simulink model "gps_estimate_pointsolution_demo"  (Simulink 7.3)
settings: Solver=ode45  StartTime=0.0  StopTime=86400  RelTol=1e-3
undefined symbols (not defined in the file): WGS
libraries: rapidstm32_gps_lib x6
settings Model: Creator=Compaq  LastModifiedBy=Compaq

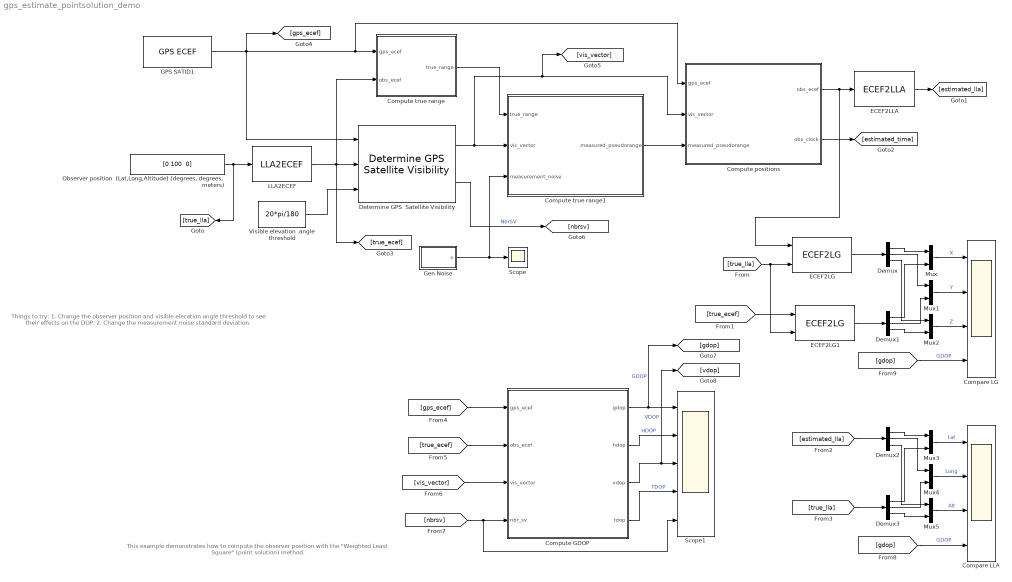
== system gps_estimate_pointsolution_demo ==
  note: This example demonstrates how to compute the observer position
      | with the "Weighted Least Square" (point solution) method.
  note: Things to try:
      | 1. Change the observer position and visible elecation angle threshold
      | to see their effects on the DOP.
      | 2. Change the measurement noise standard deviation.
  Compare LG : Scope  NumInputPorts=4
      settings: TimeRange=35000  YMin=-300~-400~-6.37925e+006~1.3  YMax=350~350~-6.377e+006~2  MaxDataPoints=1000
  Compare LLA : Scope  NumInputPorts=4
      settings: YMin=-0.00025~99.9995~-100~1.3  YMax=0.00025~100~100~1.95  SaveName=ScopeData2  MaxDataPoints=1000
  Compute GDOP : Stateflow chart
  Compute positions : Stateflow chart
  Compute true range : Stateflow chart
  Compute true range1 : Stateflow chart
  Demux{,1..3} (4 alike) : Demux  Outputs=3
  Determine GPS  Satellite Visibility : rapidstm32_gps_lib/Determine GPS  Satellite Visibility
  ECEF2LG : rapidstm32_gps_lib/ECEF2LG  lgoutput_format=NED  latlong_format=Degrees
  ECEF2LG1 : rapidstm32_gps_lib/ECEF2LG  lgoutput_format=NED  latlong_format=Degrees
  ECEF2LLA : rapidstm32_gps_lib/ECEF2LLA  latlong_format=Degrees  altitude_format=Meters  refellipsoid=WGS-84  re=6378137  epsilon=0.081819190842622
  GPS SATID1 : rapidstm32_gps_lib/GPS ECEF  satid=All 24  t0=0  sampletime=30
  Gen Noise : Stateflow chart
  LLA2ECEF : rapidstm32_gps_lib/LLA2ECEF  latlong_format=Degrees  refellipsoid=WGS-84  re=6378137  epsilon=0.081819190842622
  Mux{,1..5} (6 alike) : Mux  Inputs=2
  "Observer position  (Lat,Long,Altitude) (degrees, degrees, meters)" : Constant  Value="[0 100  0]"  OutDataType=fixdt(1, 16)  OutScaling=2^0
  Scope : Scope
      settings: YMin=-35  YMax=40  MaxDataPoints=1000
  Scope1 : Scope  NumInputPorts=5
      settings: TimeRange=86400  YMin=1~0~0~-8.67362e-019~1  YMax=8~30~25~0.03~4  SaveName=ScopeData3
  Visible elevation  angle threshold : Constant  Value=20*pi/180  OutDataType=fixdt(1, 16)  OutScaling=2^0
  wires:
  GPS SATID1/1 -> Determine GPS  Satellite Visibility/1, Compute true range/1(gps_ecef), Compute positions/1(gps_ecef), [gps_ecef]
  "Observer position  (Lat,Long,Altitude) (degrees, degrees, meters)"/1 -> LLA2ECEF/1, [true_lla]
  LLA2ECEF/1 -> Compute true range/2(obs_ecef), Determine GPS  Satellite Visibility/2, [true_ecef]
  Visible elevation  angle threshold/1 -> Determine GPS  Satellite Visibility/3
  Compute true range/1(true_range) -> Compute true range1/1(true_range)
  Determine GPS  Satellite Visibility/1 -> Compute true range1/2(vis_vector), Compute positions/2(vis_vector), [vis_vector]
  Gen Noise/1(n) -> Scope/1, Compute true range1/3(measurement_noise)
  Compute true range1/1(measured_pseudorange) -> Compute positions/3(measured_pseudorange)
  Determine GPS  Satellite Visibility/2 -> [nbrsv]  "NbrSV"
  Compute positions/1(obs_ecef) -> ECEF2LLA/1, ECEF2LG/1
  ECEF2LLA/1 -> [estimated_lla]
  Compute positions/2(obs_clock) -> [estimated_time]
  [true_lla] -> ECEF2LG/2, ECEF2LG1/2
  [true_ecef] -> ECEF2LG1/1
  ECEF2LG/1 -> Demux/1
  ECEF2LG1/1 -> Demux1/1
  Mux/1 -> Compare LG/1  "X"
  Mux1/1 -> Compare LG/2  "Y"
  Mux2/1 -> Compare LG/3  "Z"
  Demux/1 -> Mux/1
  Demux1/1 -> Mux/2
  Demux/2 -> Mux1/1
  Demux1/2 -> Mux1/2
  Demux/3 -> Mux2/1
  Demux1/3 -> Mux2/2
  Mux3/1 -> Compare LLA/1  "Lat"
  Mux4/1 -> Compare LLA/2  "Long"
  Mux5/1 -> Compare LLA/3  "Alt"
  Demux2/1 -> Mux3/1
  Demux3/1 -> Mux3/2
  Demux2/2 -> Mux4/1
  Demux3/2 -> Mux4/2
  Demux2/3 -> Mux5/1
  Demux3/3 -> Mux5/2
  [true_lla] -> Demux3/1
  [estimated_lla] -> Demux2/1
  Compute GDOP/1(gdop) -> Scope1/1, [gdop]  "GDOP"
  Compute GDOP/2(hdop) -> Scope1/2  "HDOP"
  Compute GDOP/3(vdop) -> Scope1/3, [vdop]  "VDOP"
  Compute GDOP/4(tdop) -> Scope1/4  "TDOP"
  [gps_ecef] -> Compute GDOP/1(gps_ecef)
  [true_ecef] -> Compute GDOP/2(obs_ecef)
  [vis_vector] -> Compute GDOP/3(vis_vector)
  [nbrsv] -> Compute GDOP/4(nbr_sv), Scope1/5
  [gdop] -> Compare LLA/4  "GDOP"
  [gdop] -> Compare LG/4  "GDOP"

== matlab function Compute true range1 ==
  data: true_range input double; vis_vector input double; measurement_noise input double; measured_pseudorange output double
function measured_pseudorange = f(true_range, vis_vector, measurement_noise)
%#eml

% Make true ranges into measured pseudorange by adding measurement noises.
% All measurement noises (clock drift, multipath, atmospheric delay, etc.) 
% are simply assumed to be random white noise.

nbrofsv = length(vis_vector);
measured_pseudorange = zeros(nbrofsv,1);
idx = 1;
for k = 1:nbrofsv
    if (vis_vector(k) == 1)
        measured_pseudorange(idx) = true_range(k) + measurement_noise(k);
        idx = idx + 1;
    end
end

== matlab function Compute true range ==
  data: gps_ecef input double; true_range output double; obs_ecef input double
function true_range = f(gps_ecef, obs_ecef)
%#eml

% Compute true range between the observer and each satellite
true_range = sqrt(sum((gps_ecef - repmat(obs_ecef,1,24)).^2,1));

== matlab function Compute positions ==
  data: gps_ecef input double; vis_vector input double; measured_pseudorange input double; obs_ecef output double; obs_clock output double
function [obs_ecef, obs_clock] = f(gps_ecef, vis_vector, measured_pseudorange)
%#eml

% Compute position using Weighted Least Square Method

persistent current_position

if isempty(current_position)
    %current_position = [-1.108e6 6.281e6 0];
    current_position = [6.378e6 0 0];
end

persistent current_time

if isempty(current_time)
    current_time = 0;
end

persistent firsttime

if isempty(firsttime)
    firsttime = 1;
end

% usesat = 4;
nbrofsv = length(vis_vector);
cosine_vector = zeros(nbrofsv,3);
G = zeros(nbrofsv,4);
dr = zeros(nbrofsv,1);
R = diag(100*ones(1,nbrofsv));
if firsttime 
    % Initial position estimates with iterative process to obtain the closest
    % position estimate to the true position as possible.
    for i = 1:10
        idx = 1;
        for k = 1:nbrofsv
            if (vis_vector(k) == 1)
                cosine_vector(idx,:) = gps_ecef(:,k)' - current_position;
                r_ref = sqrt(sum(cosine_vector(idx,:).^2,2)); % assuming 0 user clock offset
                G(idx,:) = [-cosine_vector(idx,:)./repmat(r_ref,1,3) 1];
                dr(idx) = measured_pseudorange(idx) - r_ref;
                idx = idx + 1;
            end
        end
        % dx = wls(G(1:usesat,:),dr(1:usesat),R(1:usesat,1:usesat));
        dx = wls(G(1:nbrofsv,:),dr(1:nbrofsv),R(1:nbrofsv,1:nbrofsv));
        current_position = current_position + dx(1:3)';
        current_time = current_time + dx(4)/3e8;
    end
    firsttime = 0;
else
    idx = 1;
    for k = 1:nbrofsv
        if (vis_vector(k) == 1)
            cosine_vector(idx,:) = gps_ecef(:,k)' - current_position;
            r_ref = sqrt(sum(cosine_vector(idx,:).^2,2)); % assuming 0 user clock offset
            G(idx,:) = [-cosine_vector(idx,:)./repmat(r_ref,1,3) 1];
            dr(idx) = measured_pseudorange(idx) - r_ref;
            idx = idx + 1;
        end
    end
    % dx = wls(G(1:usesat,:),dr(1:usesat),R(1:usesat,1:usesat));
    dx = wls(G(1:nbrofsv,:),dr(1:nbrofsv),R(1:nbrofsv,1:nbrofsv));
    current_position = current_position + dx(1:3)';
    current_time = current_time + dx(4)/3e8;
end
obs_ecef = current_position';
obs_clock = current_time;


%function [x,dx] = wls(H,y,R)
function x = wls(H,y,R)

% Weighted Least Squares estimator
%
% function [x,dx] = wls(H,y,R);
%
% calculate the least squares estimate of a system
%
% y = Hx+e
%
% H must be m-by-n where m > n
%
% y is the measurement vector
% H is the measurement matrix
% e is the measurement noise with covariance matrix R = E[eeT]
% x is the system state variables
% dx is the standard errors of x
% dx = sqrt(diag(P));
%
% This function differs from Matlab lscov in that the solution is found by inverting matrixs.
% the standard errors of x is independent of y
%
% The formula:
% xe = inv(H'*inv(R)*H)*H'*inv(R)*y
% P = inv(H'*inv(R)*H)
%
% References:
%       G. Strang, "Introduction to Applied Mathematics",
%       Wellesley-Cambridge, 1986

% method 1
% HT = H.';
% HTinvR = HT/R;
% x = (HTinvR*H)\(HTinvR)*y;
% dx = sqrt(diag(dxcov));
%
% method 2
x = H\y;

== matlab function Gen Noise ==
  data: n output double
function n = fcn
%#eml

noise_standard_deviation = 10; % measurement noise standard deviation in meters
n = randn(24,1)*noise_standard_deviation;

== matlab function Compute GDOP ==
  data: gps_ecef input double; obs_ecef input double; vis_vector input double; gdop output double; nbr_sv input double; hdop output double; vdop output double; tdop output double
function [gdop, hdop, vdop, tdop] = compute_dop(gps_ecef, obs_ecef, vis_vector, nbr_sv)
%#eml

% This algorithm is not yet optimized due to limitation of the Embedded
% MATLAB function block which does not allow for dynamic vector/matrix indexing.
% So G is still a 24-by-4 matrix even if not all satellites are visible.

G = [zeros(24,3) ones(24,1)];
idx = 1;
for i = 1:24
    if (vis_vector(i) == 1)
        unit_vector = gps_ecef(:,i) - obs_ecef;
        r = sqrt(sum(unit_vector.^2,1));
        G(idx,1:3) = -unit_vector'./r;
        idx = idx + 1;
    end
end
if (idx >= 4)
    dop = inv(G'*G); % to be optimized
    gdop = sqrt(trace(dop));
    hdop = sqrt(sum(dop(1:2).^2));
    vdop = sqrt(dop(3).^2);
    tdop = sqrt(dop(4).^2);
else
    gdop = NaN;
    hdop = NaN;
    vdop = NaN;
    tdop = NaN;
end
